simulink subsystem "const_controller"  (R2024b)
settings: Solver=VariableStepAuto  StartTime=0.0  StopTime=10.0  RelTol=1e-3
undefined symbols (not defined in the file or in its folder): const_brake
settings Model: Creator=yevge  LastModifiedBy=yevge

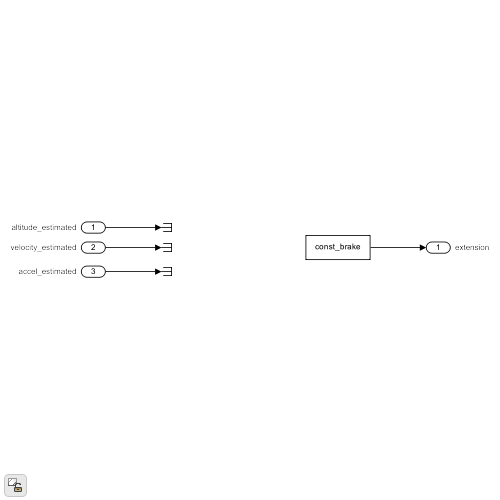
[thumbnail: Simulink's stored preview of the top-level diagram]
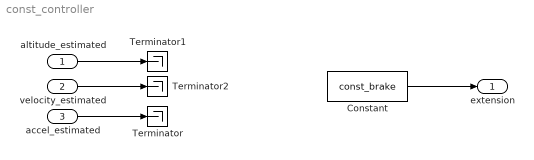
== system const_controller ==
  altitude_estimated : Inport  Unit=m  PortDimensions=1
  velocity_estimated : Inport  Port=2  Unit=m/s  PortDimensions=1
  accel_estimated : Inport  Port=3  Unit=m/s^2  PortDimensions=1
  Constant : Constant  Value=const_brake
  Terminator : Terminator
  Terminator1 : Terminator
  Terminator2 : Terminator
  extension : Outport  OutMin=0  OutMax=1  Unit=1  PortDimensions=1  InitialOutput=const_brake
  wires:
  accel_estimated/1 -> Terminator/1
  altitude_estimated/1 -> Terminator1/1
  Constant/1 -> extension/1
  velocity_estimated/1 -> Terminator2/1
